simulink model "FOCandPMSM"  (R2022b)
settings: Solver=FixedStepAuto  StartTime=0.0  StopTime=inf  RelTol=1e-3  EnableMultiTasking=on
PreLoadFcn:
  | Ts = 1e-4;
  | Tcpu = 50e-6; %Controller sample time
  | 
  | % PMSM parameters
  | PM = 0.03; % Permanent magnet flux linkage
  | Ld = 2e-4;  % d-axis inductance
  | Lq = 2e-4;  % q-axis inductance
  | L0 = 2e-4;  % 0-axis inductance
  | Rs = 0.013; % Stator resistance
  | N = 6; % Number of pole pairs
  | J = 0.2; % Moment of inertia
  | 
  | % encoder parameters
  | numSlits = 2000; % number of slits
  | pulseSigOffset = 0; % index pulse signal offset
  | shaftInitPos = 0; % motor shaft initial position
  | 
  | % DAC parameters
  | gain = 0.1;
  | bias = 0;
  | 
  | % circuit parameters
  | Vdc = 48;
  | 
  | % real-time parameters
  | ts_FPGA_clk = 5e-9;
  | ts_FPGA_mdl = 1e-6;
  | 
  | % Real-time processor or embedded controller
  | RTorTTL = 1; % 1: Real-time processor,    0: embedded controller
  | 
  | % sample times
  | f_base = 200e6;
  | PWM_frequency = 20e3;
  | ts_FPGA_clk = 1/f_base;
  | ts_FPGA_mdl =1e-6;
  | 
  | PMSM_HIL_Param;
values from neighbouring files (symbols this model uses):
  inverter = mcb_updateInverterParameters(pmsm,inverter,target)    [embedded_sim_codegen_data.m]
  pmsm = mcb_SetPMSMMotorParameters('Teknic2310P')    [embedded_sim_codegen_data.m]
  PU_System = mcb_SetPUSystem(pmsm,inverter)    [embedded_sim_codegen_data.m]
  SpeedRef = 1    [PMSM_HIL_Param.m]
  T_cpu = T_pwm    (= 5e-05)    [embedded_sim_codegen_data.m]
  Tsw = 1/f_sw    [PMSM_HIL_Param.m]
undefined symbols (not defined in the file or in its folder): IO334
libraries: speedgoatlib_hdlCoder_IO3xx x28, mcbpositiondecoderlib x2, mcbhdlplantlib x1, slrtencoderlib x1, slrtresolverlib x1, mcbcontrolslib x1
settings Model: Creator=chrisz  LastModifiedBy=chrisz
settings SolverCC: ConcurrentTasks=on  PositivePriorityOrder=on
settings OptimizationCC: BlockReduction=off  ConditionallyExecuteInputs=off  OptimizeBlockIOStorage=off
settings DebuggingCC: AlgebraicLoopMsg=error  InheritedTsInSrcMsg=none  SingleTaskRateTransMsg=error  TasksWithSamePriorityMsg=none  ParameterOverflowMsg=none  ParameterUnderflowMsg=error  ParameterPrecisionLossMsg=none  InheritVATfromSVC=none  VariantConfigNotUsedByTopModel=none
settings HardwareCC: ProdBitPerLong=64  ProdLongLongMode=on  ProdHWDeviceType=Intel->x86-64 (Linux 64)  TargetBitPerPointer=64  TargetBitPerSizeT=64  TargetBitPerPtrDiffT=64  TargetLongLongMode=on  TargetIntDivRoundTo=Zero  TargetEndianess=LittleEndian  TargetWordSize=64  TargetHWDeviceType=Custom Processor->MATLAB Host Computer
settings ModelReferenceCC: EnableRefExpFcnMdlSchedulingChecks=on
settings RTWCC: Description=Simulink Real-Time  SystemTargetFile=slrealtime.tlc  TemplateMakefile=slrealtime_default_tmf  Toolchain=Simulink Real-Time Toolchain  BuildConfiguration=Faster Runs  CodeExecutionProfiling=on  TargetLang=C++

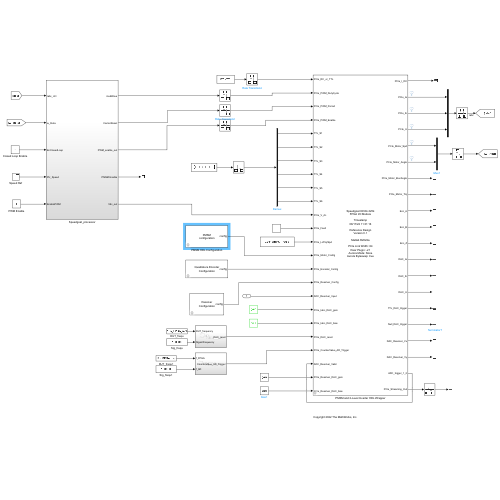
[thumbnail: Simulink's stored preview of the top-level diagram]
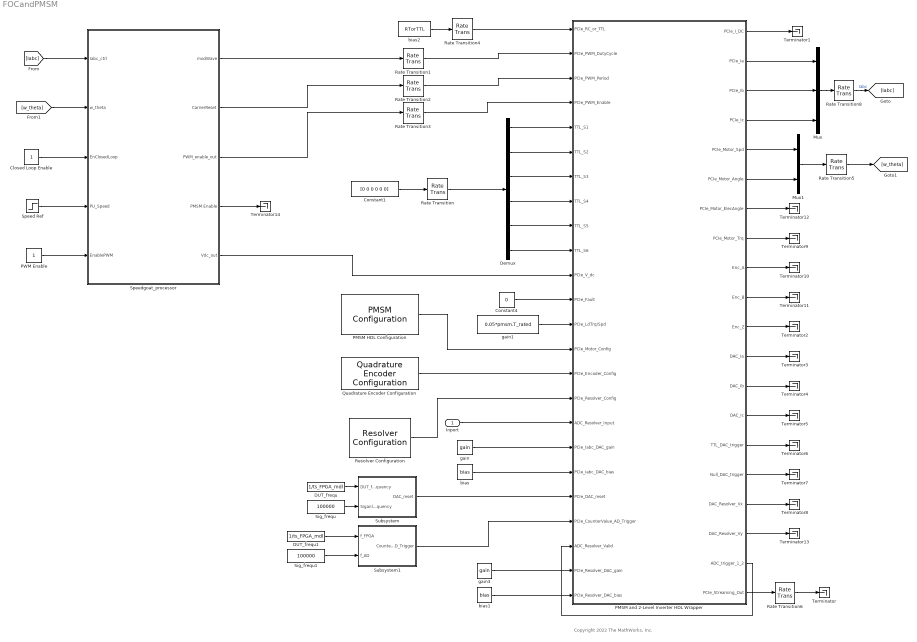
== system FOCandPMSM ==
  note: Copyright 2022 The MathWorks, Inc.
  Inport : Inport  OutDataTypeStr=int16
  Closed Loop Enable : Constant  OutDataTypeStr=Inherit: Inherit via back propagation  SampleTime=-1
  Constant1 : Constant  Value=[0 0 0 0 0 0]  OutDataTypeStr=boolean  SampleTime=-1
  Constant4 : Constant  Value=0  OutDataTypeStr=uint32  SampleTime=Tcpu
  DUT_frequ : Constant  Value=1/ts_FPGA_mdl  SampleTime=Tcpu
  DUT_frequ1 : Constant  Value=1/ts_FPGA_mdl  SampleTime=Tcpu
  Demux : Demux  Outputs=6
  Mux : Mux  Inputs=3
  Mux1 : Mux  Inputs=2
  PMSM HDL Configuration : mcbhdlplantlib/PMSM Configuration  portConfig=Torque  Trq_N_mode=0  Ts=Tcpu  Pp=pmsm.p  Rs=pmsm.Rs  Ld=pmsm.Ld  Lq=pmsm.Lq  lambda_pm=pmsm.FluxPM  J=pmsm.J  B=pmsm.B  f=0
      settings: LibrarySourceBlock=mcbhdllib/Electrical Systems/Motors/PMSM Configuration
  PMSM and 2-Level Inverter HDL Wrapper : Subsystem  mask(Speedgoat IO334-325k Interface Block){module_id=1, slot=-1, ts=-1, OutputRange=Auto (same as ADC), PullRPort0=pull-down, VioPort0=3.3V, PullRPort1=pull-down, VioPort1=3.3V, PullRPort2=pull-down, VioPort2=3.3V, PullRPort3=pull-down, VioPort3=3.3V, PullRPort4=pull-down, VioPort4=3.3V, PullRPort5=pull-down, VioPort5=3.3V, PullRPort6=pull-down, VioPort6=3.3V, FpgaFreq=200}
      mask prompts: module_id "FPGA Module Identifier:"; slot "PCI slot (-1: autosearch):"; ts "Sample time:"; OutputRange "DAC Voltage Range:"; PullRPort0 "pull resistor"; VioPort0 "I/O voltage"; PullRPort1 "pull resistor"; VioPort1 "I/O voltage"; PullRPort2 "pull resistor"; VioPort2 "I/O voltage"; PullRPort3 "pull resistor"; VioPort3 "I/O voltage"; PullRPort4 "pull resistor"; VioPort4 "I/O voltage"; PullRPort5 "pull resistor"; VioPort5 "I/O voltage"; PullRPort6 "pull resistor"; VioPort6 "I/O voltage"; FpgaFreq "FPGA Frequency [MHz]"
      mask help: Simulink Real-Time Interface Block for Speedgoat IO334-325k.
      mask init:
      | hdlslrt.backend.mfpgaparameters;
      mask Help: eval('speedgoatdoc_hdlc')
      mask TypeOptions OutputRange: IO334 DAC Setup/OutputRange
      mask TypeOptions PullRPort0: Port Settings -2x/PullRPort0
      mask Callback PullRPort0: sg_fpga_HDLCoder_io3xx_2x_m(2)
      mask TypeOptions VioPort0: Port Settings -2x/VioPort0
      mask Callback VioPort0: sg_fpga_HDLCoder_io3xx_2x_m(2)
      mask TypeOptions PullRPort1: Port Settings -2x/PullRPort1
      mask Callback PullRPort1: sg_fpga_HDLCoder_io3xx_2x_m(2)
      mask TypeOptions VioPort1: Port Settings -2x/VioPort1
      mask Callback VioPort1: sg_fpga_HDLCoder_io3xx_2x_m(2)
      mask TypeOptions PullRPort2: Port Settings -2x/PullRPort2
      mask Callback PullRPort2: sg_fpga_HDLCoder_io3xx_2x_m(2)
      mask TypeOptions VioPort2: Port Settings -2x/VioPort2
      mask Callback VioPort2: sg_fpga_HDLCoder_io3xx_2x_m(2)
      mask TypeOptions PullRPort3: Port Settings -2x/PullRPort3
      mask Callback PullRPort3: sg_fpga_HDLCoder_io3xx_2x_m(2)
      mask TypeOptions VioPort3: Port Settings -2x/VioPort3
      mask Callback VioPort3: sg_fpga_HDLCoder_io3xx_2x_m(2)
      mask TypeOptions PullRPort4: Port Settings -2x/PullRPort4
      mask Callback PullRPort4: sg_fpga_HDLCoder_io3xx_2x_m(2)
      mask TypeOptions VioPort4: Port Settings -2x/VioPort4
      mask Callback VioPort4: sg_fpga_HDLCoder_io3xx_2x_m(2)
      mask TypeOptions PullRPort5: Port Settings -2x/PullRPort5
      mask Callback PullRPort5: sg_fpga_HDLCoder_io3xx_2x_m(2)
      mask TypeOptions VioPort5: Port Settings -2x/VioPort5
      mask Callback VioPort5: sg_fpga_HDLCoder_io3xx_2x_m(2)
      mask TypeOptions PullRPort6: Port Settings -2x/PullRPort6
      mask Callback PullRPort6: sg_fpga_HDLCoder_io3xx_2x_m(2)
      mask TypeOptions VioPort6: Port Settings -2x/VioPort6
      mask Callback VioPort6: sg_fpga_HDLCoder_io3xx_2x_m(2)
      mask DialogControl AnalogOutput Prompt: Analog Output
      mask DialogControl IO33421 Prompt: IO334-21
      mask DialogControl port1 Prompt: Port 1
      mask DialogControl port2 Prompt: Port 2
      mask DialogControl port3 Prompt: Port 3
      mask DialogControl port4 Prompt: Port 4
      mask DialogControl port5 Prompt: Port 5
      mask DialogControl port6 Prompt: Port 6
      mask DialogControl port7 Prompt: Port 7
      mask Display:
      | SetupBlkPath = find_system(gcb, 'LookUnderMasks', 'all', 'FollowLinks', 'on', 'regexp', 'on', 'Name', 'IO3(\d|x){2}\s+Setup' );
      | SetupBlkPath = SetupBlkPath{1};
      | TS = get_param(SetupBlkPath,'timestamp_mcs');
      | disp(sprintf('Speedgoat IO334-325k\nFPGA I/O Module\n\nTimestamp\n%s\n\nReference Design\nVersion 0.1\n\nMatlab R2022a\n\nPCIe Link Width: X4\nRear Plugin: -21\nAurora Mode: None\nAurora Byteswap: true\n', TS))
  PWM Enable : Constant  OutDataTypeStr=Inherit: Inherit via back propagation  SampleTime=-1
  Quadrature Encoder Configuration : slrtencoderlib/Quadrature Encoder Configuration  NPulses=2000  zOffset=0  Ts=Tcpu
  Rate Transition{,1..6,8} (8 alike) : RateTransition  OutPortSampleTime=Tcpu
  Resolver Configuration : slrtresolverlib/Resolver Configuration  Ts=Tcpu  R=0.5  N=1  ADCrefV=5  ADCbits=16  totalADCCounts=65536
  Sig_frequ : Constant  Value=100000  VectorParams1D=off  SampleTime=Tcpu
  Sig_frequ1 : Constant  Value=100000  VectorParams1D=off  SampleTime=Tcpu
  Speed Ref : Step  Time=0.25  Before=1500/PU_System.N_base  After=SpeedRef  OutDataTypeStr=dataType  SampleTime=T_cpu
  Speedgoat_processor : Subsystem
  Subsystem : Subsystem
  Subsystem1 : Subsystem
  Terminator{,1..14} (15 alike) : Terminator
  bias : Constant  Value=bias  OutDataTypeStr=single  SampleTime=Tcpu
  bias1 : Constant  Value=bias  OutDataTypeStr=single  SampleTime=Tcpu
  bias2 : Constant  Value=RTorTTL  OutDataTypeStr=single  SampleTime=Tcpu
  gain : Constant  Value=gain  OutDataTypeStr=single  SampleTime=Tcpu
  gain1 : Constant  Value=0.05*pmsm.T_rated  OutDataTypeStr=single  SampleTime=Tcpu
  gain3 : Constant  Value=gain  OutDataTypeStr=single  SampleTime=Tcpu
  wires:
  bias1/1 -> PMSM and 2-Level Inverter HDL Wrapper/24(PCIe_Resolver_DAC_bias)
  gain3/1 -> PMSM and 2-Level Inverter HDL Wrapper/23(PCIe_Resolver_DAC_gain)
  Speedgoat_processor/1(modWave) -> Rate Transition1/1
  Rate Transition5/1 -> [w_theta]
  Mux1/1 -> Rate Transition5/1
  Rate Transition8/1 -> [Iabc]  "Iabc"
  Mux/1 -> Rate Transition8/1
  Rate Transition6/1 -> Terminator/1
  DUT_frequ1/1 -> Subsystem1/1(f_FPGA)
  Sig_frequ1/1 -> Subsystem1/2(f_AD)
  PMSM and 2-Level Inverter HDL Wrapper/19(ADC_trigger_1_2) -> PMSM and 2-Level Inverter HDL Wrapper/22(ADC_Resolver_Valid)
  Subsystem1/1(CounterValue_AD_Trigger) -> PMSM and 2-Level Inverter HDL Wrapper/21(PCIe_CounterValue_AD_Trigger)
  PMSM HDL Configuration/1 -> PMSM and 2-Level Inverter HDL Wrapper/14(PCIe_Motor_Config)
  Sig_frequ/1 -> Subsystem/2(SiganlFrequency)
  DUT_frequ/1 -> Subsystem/1(DUT_frequency)
  Constant1/1 -> Rate Transition/1
  Rate Transition/1 -> Demux/1
  bias2/1 -> Rate Transition4/1
  Speed Ref/1 -> Speedgoat_processor/4(PU_Speed)
  Closed Loop Enable/1 -> Speedgoat_processor/3(EnClosedLoop)
  PWM Enable/1 -> Speedgoat_processor/5(EnablePWM)
  [w_theta] -> Speedgoat_processor/2(w_theta)
  [Iabc] -> Speedgoat_processor/1(Iabc_ctrl)
  Speedgoat_processor/2(CarrierReset) -> Rate Transition2/1
  Speedgoat_processor/3(PWM_enable_out) -> Rate Transition3/1
  Speedgoat_processor/5(Vdc_out) -> PMSM and 2-Level Inverter HDL Wrapper/11(PCIe_V_dc)
  gain1/1 -> PMSM and 2-Level Inverter HDL Wrapper/13(PCIe_LdTrq/Spd)
  bias/1 -> PMSM and 2-Level Inverter HDL Wrapper/19(PCIe_Iabc_DAC_bias)
  Subsystem/1(DAC_reset) -> PMSM and 2-Level Inverter HDL Wrapper/20(PCIe_DAC_reset)
  Speedgoat_processor/4(PMSM Enable) -> Terminator14/1
  PMSM and 2-Level Inverter HDL Wrapper/20(PCIe_Streaming_Out) -> Rate Transition6/1
  PMSM and 2-Level Inverter HDL Wrapper/18(DAC_Resolver_Vy) -> Terminator13/1
  PMSM and 2-Level Inverter HDL Wrapper/17(DAC_Resolver_Vx) -> Terminator8/1
  PMSM and 2-Level Inverter HDL Wrapper/16(Null_DAC_trigger) -> Terminator7/1
  PMSM and 2-Level Inverter HDL Wrapper/15(TTL_DAC_trigger) -> Terminator6/1
  PMSM and 2-Level Inverter HDL Wrapper/14(DAC_Ic) -> Terminator5/1
  PMSM and 2-Level Inverter HDL Wrapper/1(PCIe_I_DC) -> Terminator1/1
  PMSM and 2-Level Inverter HDL Wrapper/2(PCIe_Ia) -> Mux/1
  PMSM and 2-Level Inverter HDL Wrapper/3(PCIe_Ib) -> Mux/2
  PMSM and 2-Level Inverter HDL Wrapper/4(PCIe_Ic) -> Mux/3
  PMSM and 2-Level Inverter HDL Wrapper/5(PCIe_Motor_Spd) -> Mux1/1
  PMSM and 2-Level Inverter HDL Wrapper/6(PCIe_Motor_Angle) -> Mux1/2
  PMSM and 2-Level Inverter HDL Wrapper/7(PCIe_Motor_ElecAngle) -> Terminator12/1
  PMSM and 2-Level Inverter HDL Wrapper/8(PCIe_Motor_Trq) -> Terminator9/1
  PMSM and 2-Level Inverter HDL Wrapper/9(Enc_A) -> Terminator10/1
  PMSM and 2-Level Inverter HDL Wrapper/10(Enc_B) -> Terminator11/1
  PMSM and 2-Level Inverter HDL Wrapper/11(Enc_Z) -> Terminator2/1
  PMSM and 2-Level Inverter HDL Wrapper/12(DAC_Ia) -> Terminator3/1
  PMSM and 2-Level Inverter HDL Wrapper/13(DAC_Ib) -> Terminator4/1
  Rate Transition4/1 -> PMSM and 2-Level Inverter HDL Wrapper/1(PCIe_RC_or_TTL)
  Rate Transition1/1 -> PMSM and 2-Level Inverter HDL Wrapper/2(PCIe_PWM_DutyCycle)
  Rate Transition2/1 -> PMSM and 2-Level Inverter HDL Wrapper/3(PCIe_PWM_Period)
  Rate Transition3/1 -> PMSM and 2-Level Inverter HDL Wrapper/4(PCIe_PWM_Enable)
  Demux/1 -> PMSM and 2-Level Inverter HDL Wrapper/5(TTL_S1)
  Demux/2 -> PMSM and 2-Level Inverter HDL Wrapper/6(TTL_S2)
  Demux/3 -> PMSM and 2-Level Inverter HDL Wrapper/7(TTL_S3)
  Demux/4 -> PMSM and 2-Level Inverter HDL Wrapper/8(TTL_S4)
  Demux/5 -> PMSM and 2-Level Inverter HDL Wrapper/9(TTL_S5)
  Demux/6 -> PMSM and 2-Level Inverter HDL Wrapper/10(TTL_S6)
  Constant4/1 -> PMSM and 2-Level Inverter HDL Wrapper/12(PCIe_Fault)
  Quadrature Encoder Configuration/1 -> PMSM and 2-Level Inverter HDL Wrapper/15(PCIe_Encoder_Config)
  Resolver Configuration/1 -> PMSM and 2-Level Inverter HDL Wrapper/16(PCIe_Resolver_Config)
  Inport/1 -> PMSM and 2-Level Inverter HDL Wrapper/17(ADC_Resolver_Input)
  gain/1 -> PMSM and 2-Level Inverter HDL Wrapper/18(PCIe_Iabc_DAC_gain)

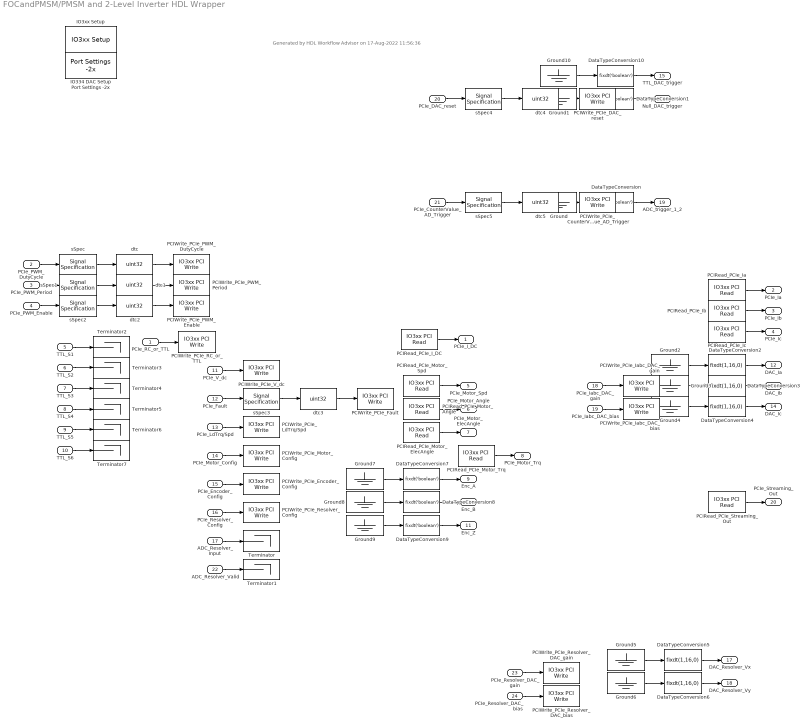
== system FOCandPMSM/PMSM and 2-Level Inverter HDL Wrapper ==
  note: Generated by HDL Workflow Advisor on 17-Aug-2022 11:56:36
  PCIe_RC_or_TTL : Inport
  PCIe_PWM_DutyCycle : Inport  Port=2
  PCIe_PWM_Period : Inport  Port=3
  PCIe_PWM_Enable : Inport  Port=4
  TTL_S1 : Inport  Port=5
  TTL_S2 : Inport  Port=6
  TTL_S3 : Inport  Port=7
  TTL_S4 : Inport  Port=8
  TTL_S5 : Inport  Port=9
  TTL_S6 : Inport  Port=10
  PCIe_V_dc : Inport  Port=11
  PCIe_Fault : Inport  Port=12
  PCIe_LdTrq/Spd : Inport  Port=13
  PCIe_Motor_Config : Inport  Port=14
  PCIe_Encoder_Config : Inport  Port=15
  PCIe_Resolver_Config : Inport  Port=16
  ADC_Resolver_Input : Inport  Port=17
  PCIe_Iabc_DAC_gain : Inport  Port=18
  PCIe_Iabc_DAC_bias : Inport  Port=19
  PCIe_DAC_reset : Inport  Port=20
  PCIe_CounterValue_AD_Trigger : Inport  Port=21  OutDataTypeStr=uint32
  ADC_Resolver_Valid : Inport  Port=22
  PCIe_Resolver_DAC_gain : Inport  Port=23
  PCIe_Resolver_DAC_bias : Inport  Port=24
  DataTypeConversion{,1,7..10} (6 alike) : DataTypeConversion  OutDataTypeStr=fixdt('boolean')  ConvertRealWorld=Stored Integer (SI)  SaturateOnIntegerOverflow=off  RndMeth=Floor
  DataTypeConversion{2..6} (5 alike) : DataTypeConversion  OutDataTypeStr=fixdt(1,16,0)  ConvertRealWorld=Stored Integer (SI)  SaturateOnIntegerOverflow=off  RndMeth=Floor
  Ground{,1..10} (11 alike) : Ground
  IO334 DAC Setup : speedgoatlib_hdlCoder_IO3xx/IO334 DAC Setup  module_id=module_id  OutputRange=Auto (same as ADC)
  IO3xx Setup : speedgoatlib_hdlCoder_IO3xx/IO3xx Setup  mdl_ss_name=slrt_pmsm_2level_inverterFrom22b/PMSM and 2-Level Inverter HDL Wrapper  board_type=IO334-325k  fpga_sync_mode=on  reset_mode=on  reset_mode_stop=off  device_id=1  module_id=module_id  pci_slot=slot  fpga_mat_file=hdl_prj\hdlsrc\slrt_pmsm_2level_inverterFrom22b\PMSMAnd2_LevelInverterHDLWrapper.mat  timestamp_mcs=08/17/22 11:31:16  timestamp=2208171019  tsreg=hex2dec('8')  bsf_file=PMSMAnd2_LevelInverterHDLWrapper.mcs  mcs=0
  PCIRead_PCIe_I_DC : speedgoatlib_hdlCoder_IO3xx/IO3xx PCI Read  device_id=1  module_id=module_id  board_type=IO334-325k  port_name=PCIe_I_DC  port_offset=hex2dec('184')  port_type=single  port_dim=1  strobe=0  sample_time=ts
  PCIRead_PCIe_Ia : speedgoatlib_hdlCoder_IO3xx/IO3xx PCI Read  device_id=1  module_id=module_id  board_type=IO334-325k  port_name=PCIe_Ia  port_offset=hex2dec('188')  port_type=single  port_dim=1  strobe=0  sample_time=ts
  PCIRead_PCIe_Ib : speedgoatlib_hdlCoder_IO3xx/IO3xx PCI Read  device_id=1  module_id=module_id  board_type=IO334-325k  port_name=PCIe_Ib  port_offset=hex2dec('18C')  port_type=single  port_dim=1  strobe=0  sample_time=ts
  PCIRead_PCIe_Ic : speedgoatlib_hdlCoder_IO3xx/IO3xx PCI Read  device_id=1  module_id=module_id  board_type=IO334-325k  port_name=PCIe_Ic  port_offset=hex2dec('1A4')  port_type=single  port_dim=1  strobe=0  sample_time=ts
  PCIRead_PCIe_Motor_Angle : speedgoatlib_hdlCoder_IO3xx/IO3xx PCI Read  device_id=1  module_id=module_id  board_type=IO334-325k  port_name=PCIe_Motor_Angle  port_offset=hex2dec('1AC')  port_type=single  port_dim=1  strobe=0  sample_time=ts
  PCIRead_PCIe_Motor_ElecAngle : speedgoatlib_hdlCoder_IO3xx/IO3xx PCI Read  device_id=1  module_id=module_id  board_type=IO334-325k  port_name=PCIe_Motor_ElecAngle  port_offset=hex2dec('1B0')  port_type=single  port_dim=1  strobe=0  sample_time=ts
  PCIRead_PCIe_Motor_Spd : speedgoatlib_hdlCoder_IO3xx/IO3xx PCI Read  device_id=1  module_id=module_id  board_type=IO334-325k  port_name=PCIe_Motor_Spd  port_offset=hex2dec('1A8')  port_type=single  port_dim=1  strobe=0  sample_time=ts
  PCIRead_PCIe_Motor_Trq : speedgoatlib_hdlCoder_IO3xx/IO3xx PCI Read  device_id=1  module_id=module_id  board_type=IO334-325k  port_name=PCIe_Motor_Trq  port_offset=hex2dec('124')  port_type=single  port_dim=1  strobe=0  sample_time=ts
  PCIRead_PCIe_Streaming_Out : speedgoatlib_hdlCoder_IO3xx/IO3xx PCI Read  device_id=1  module_id=module_id  board_type=IO334-325k  port_name=PCIe_Streaming_Out  port_offset=hex2dec('800')  port_type=single  port_dim=150  strobe=hex2dec('C00')  sample_time=ts
  PCIWrite_PCIe_CounterValue_AD_Trigger : speedgoatlib_hdlCoder_IO3xx/IO3xx PCI Write  device_id=1  module_id=module_id  board_type=IO334-325k  port_name=PCIe_CounterValue_AD_Trigger  port_offset=hex2dec('13C')  port_type=uint32  port_dim=1  strobe=0  sample_time=ts
  PCIWrite_PCIe_DAC_reset : speedgoatlib_hdlCoder_IO3xx/IO3xx PCI Write  device_id=1  module_id=module_id  board_type=IO334-325k  port_name=PCIe_DAC_reset  port_offset=hex2dec('138')  port_type=uint32  port_dim=1  strobe=0  sample_time=ts
  PCIWrite_PCIe_Encoder_Config : speedgoatlib_hdlCoder_IO3xx/IO3xx PCI Write  device_id=1  module_id=module_id  board_type=IO334-325k  port_name=PCIe_Encoder_Config  port_offset=hex2dec('190')  port_type=single  port_dim=3  strobe=hex2dec('1A0')  sample_time=ts
  PCIWrite_PCIe_Fault : speedgoatlib_hdlCoder_IO3xx/IO3xx PCI Write  device_id=1  module_id=module_id  board_type=IO334-325k  port_name=PCIe_Fault  port_offset=hex2dec('128')  port_type=uint32  port_dim=1  strobe=0  sample_time=ts
  PCIWrite_PCIe_Iabc_DAC_bias : speedgoatlib_hdlCoder_IO3xx/IO3xx PCI Write  device_id=1  module_id=module_id  board_type=IO334-325k  port_name=PCIe_Iabc_DAC_bias  port_offset=hex2dec('134')  port_type=single  port_dim=1  strobe=0  sample_time=ts
  PCIWrite_PCIe_Iabc_DAC_gain : speedgoatlib_hdlCoder_IO3xx/IO3xx PCI Write  device_id=1  module_id=module_id  board_type=IO334-325k  port_name=PCIe_Iabc_DAC_gain  port_offset=hex2dec('130')  port_type=single  port_dim=1  strobe=0  sample_time=ts
  PCIWrite_PCIe_LdTrq/Spd : speedgoatlib_hdlCoder_IO3xx/IO3xx PCI Write  device_id=1  module_id=module_id  board_type=IO334-325k  port_name=PCIe_LdTrq//Spd  port_offset=hex2dec('12C')  port_type=single  port_dim=1  strobe=0  sample_time=ts
  PCIWrite_PCIe_Motor_Config : speedgoatlib_hdlCoder_IO3xx/IO3xx PCI Write  device_id=1  module_id=module_id  board_type=IO334-325k  port_name=PCIe_Motor_Config  port_offset=hex2dec('140')  port_type=single  port_dim=9  strobe=hex2dec('180')  sample_time=ts
  PCIWrite_PCIe_PWM_DutyCycle : speedgoatlib_hdlCoder_IO3xx/IO3xx PCI Write  device_id=1  module_id=module_id  board_type=IO334-325k  port_name=PCIe_PWM_DutyCycle  port_offset=hex2dec('110')  port_type=uint32  port_dim=3  strobe=hex2dec('120')  sample_time=ts
  PCIWrite_PCIe_PWM_Enable : speedgoatlib_hdlCoder_IO3xx/IO3xx PCI Write  device_id=1  module_id=module_id  board_type=IO334-325k  port_name=PCIe_PWM_Enable  port_offset=hex2dec('108')  port_type=uint32  port_dim=1  strobe=0  sample_time=ts
  PCIWrite_PCIe_PWM_Period : speedgoatlib_hdlCoder_IO3xx/IO3xx PCI Write  device_id=1  module_id=module_id  board_type=IO334-325k  port_name=PCIe_PWM_Period  port_offset=hex2dec('104')  port_type=uint32  port_dim=1  strobe=0  sample_time=ts
  PCIWrite_PCIe_RC_or_TTL : speedgoatlib_hdlCoder_IO3xx/IO3xx PCI Write  device_id=1  module_id=module_id  board_type=IO334-325k  port_name=PCIe_RC_or_TTL  port_offset=hex2dec('100')  port_type=single  port_dim=1  strobe=0  sample_time=ts
  PCIWrite_PCIe_Resolver_Config : speedgoatlib_hdlCoder_IO3xx/IO3xx PCI Write  device_id=1  module_id=module_id  board_type=IO334-325k  port_name=PCIe_Resolver_Config  port_offset=hex2dec('1C0')  port_type=single  port_dim=6  strobe=hex2dec('1E0')  sample_time=ts
  PCIWrite_PCIe_Resolver_DAC_bias : speedgoatlib_hdlCoder_IO3xx/IO3xx PCI Write  device_id=1  module_id=module_id  board_type=IO334-325k  port_name=PCIe_Resolver_DAC_bias  port_offset=hex2dec('1B8')  port_type=single  port_dim=1  strobe=0  sample_time=ts
  PCIWrite_PCIe_Resolver_DAC_gain : speedgoatlib_hdlCoder_IO3xx/IO3xx PCI Write  device_id=1  module_id=module_id  board_type=IO334-325k  port_name=PCIe_Resolver_DAC_gain  port_offset=hex2dec('1B4')  port_type=single  port_dim=1  strobe=0  sample_time=ts
  PCIWrite_PCIe_V_dc : speedgoatlib_hdlCoder_IO3xx/IO3xx PCI Write  device_id=1  module_id=module_id  board_type=IO334-325k  port_name=PCIe_V_dc  port_offset=hex2dec('10C')  port_type=single  port_dim=1  strobe=0  sample_time=ts
  Port Settings -2x : speedgoatlib_hdlCoder_IO3xx/Port Settings -2x  module_id=module_id  rearIO=-21  PullRPort0=pull-down  VioPort0=3.3V  PullRPort1=pull-down  VioPort1=3.3V  PullRPort2=pull-down  VioPort2=3.3V  PullRPort3=pull-down  VioPort3=3.3V  PullRPort4=pull-down  VioPort4=3.3V  PullRPort5=pull-down  VioPort5=3.3V  PullRPort6=pull-down  VioPort6=3.3V
  Terminator{,1..7} (8 alike) : Terminator
  dtc{,1..5} (6 alike) : DataTypeConversion  OutDataTypeStr=uint32  ConvertRealWorld=Stored Integer (SI)  SaturateOnIntegerOverflow=off
  sSpec{,1,3,5} (4 alike) : SignalSpecification  OutDataTypeStr=fixdt(0,32,0)
  sSpec2 : SignalSpecification  OutDataTypeStr=fixdt('boolean')
  sSpec4 : SignalSpecification  OutDataTypeStr=fixdt(0,16,0)
  PCIe_I_DC : Outport
  PCIe_Ia : Outport  Port=2
  PCIe_Ib : Outport  Port=3
  PCIe_Ic : Outport  Port=4
  PCIe_Motor_Spd : Outport  Port=5
  PCIe_Motor_Angle : Outport  Port=6
  PCIe_Motor_ElecAngle : Outport  Port=7
  PCIe_Motor_Trq : Outport  Port=8
  Enc_A : Outport  Port=9
  Enc_B : Outport  Port=10
  Enc_Z : Outport  Port=11
  DAC_Ia : Outport  Port=12
  DAC_Ib : Outport  Port=13
  DAC_Ic : Outport  Port=14
  TTL_DAC_trigger : Outport  Port=15
  Null_DAC_trigger : Outport  Port=16
  DAC_Resolver_Vx : Outport  Port=17
  DAC_Resolver_Vy : Outport  Port=18
  ADC_trigger_1_2 : Outport  Port=19  OutDataTypeStr=boolean
  PCIe_Streaming_Out : Outport  Port=20
  wires:
  PCIe_RC_or_TTL/1 -> PCIWrite_PCIe_RC_or_TTL/1
  PCIe_PWM_DutyCycle/1 -> sSpec/1
  sSpec/1 -> dtc/1
  dtc/1 -> PCIWrite_PCIe_PWM_DutyCycle/1
  PCIe_PWM_Period/1 -> sSpec1/1
  sSpec1/1 -> dtc1/1
  dtc1/1 -> PCIWrite_PCIe_PWM_Period/1
  PCIe_PWM_Enable/1 -> sSpec2/1
  sSpec2/1 -> dtc2/1
  dtc2/1 -> PCIWrite_PCIe_PWM_Enable/1
  PCIe_V_dc/1 -> PCIWrite_PCIe_V_dc/1
  PCIe_Fault/1 -> sSpec3/1
  sSpec3/1 -> dtc3/1
  dtc3/1 -> PCIWrite_PCIe_Fault/1
  PCIe_LdTrq/Spd/1 -> PCIWrite_PCIe_LdTrq/Spd/1
  PCIe_Motor_Config/1 -> PCIWrite_PCIe_Motor_Config/1
  PCIe_Encoder_Config/1 -> PCIWrite_PCIe_Encoder_Config/1
  PCIe_Resolver_Config/1 -> PCIWrite_PCIe_Resolver_Config/1
  PCIe_Iabc_DAC_gain/1 -> PCIWrite_PCIe_Iabc_DAC_gain/1
  PCIe_Iabc_DAC_bias/1 -> PCIWrite_PCIe_Iabc_DAC_bias/1
  PCIe_DAC_reset/1 -> sSpec4/1
  sSpec4/1 -> dtc4/1
  dtc4/1 -> PCIWrite_PCIe_DAC_reset/1
  PCIe_CounterValue_AD_Trigger/1 -> sSpec5/1
  sSpec5/1 -> dtc5/1
  dtc5/1 -> PCIWrite_PCIe_CounterValue_AD_Trigger/1
  PCIe_Resolver_DAC_gain/1 -> PCIWrite_PCIe_Resolver_DAC_gain/1
  PCIe_Resolver_DAC_bias/1 -> PCIWrite_PCIe_Resolver_DAC_bias/1
  PCIRead_PCIe_I_DC/1 -> PCIe_I_DC/1
  PCIRead_PCIe_Ia/1 -> PCIe_Ia/1
  PCIRead_PCIe_Ib/1 -> PCIe_Ib/1
  PCIRead_PCIe_Ic/1 -> PCIe_Ic/1
  PCIRead_PCIe_Motor_Spd/1 -> PCIe_Motor_Spd/1
  PCIRead_PCIe_Motor_Angle/1 -> PCIe_Motor_Angle/1
  PCIRead_PCIe_Motor_ElecAngle/1 -> PCIe_Motor_ElecAngle/1
  PCIRead_PCIe_Motor_Trq/1 -> PCIe_Motor_Trq/1
  PCIRead_PCIe_Streaming_Out/1 -> PCIe_Streaming_Out/1
  ADC_Resolver_Input/1 -> Terminator/1
  ADC_Resolver_Valid/1 -> Terminator1/1
  DataTypeConversion/1 -> ADC_trigger_1_2/1
  Ground/1 -> DataTypeConversion/1
  DataTypeConversion1/1 -> Null_DAC_trigger/1
  Ground1/1 -> DataTypeConversion1/1
  DataTypeConversion2/1 -> DAC_Ia/1
  Ground2/1 -> DataTypeConversion2/1
  DataTypeConversion3/1 -> DAC_Ib/1
  Ground3/1 -> DataTypeConversion3/1
  DataTypeConversion4/1 -> DAC_Ic/1
  Ground4/1 -> DataTypeConversion4/1
  DataTypeConversion5/1 -> DAC_Resolver_Vx/1
  Ground5/1 -> DataTypeConversion5/1
  DataTypeConversion6/1 -> DAC_Resolver_Vy/1
  Ground6/1 -> DataTypeConversion6/1
  TTL_S1/1 -> Terminator2/1
  TTL_S2/1 -> Terminator3/1
  TTL_S3/1 -> Terminator4/1
  TTL_S4/1 -> Terminator5/1
  TTL_S5/1 -> Terminator6/1
  TTL_S6/1 -> Terminator7/1
  DataTypeConversion7/1 -> Enc_A/1
  Ground7/1 -> DataTypeConversion7/1
  DataTypeConversion8/1 -> Enc_B/1
  Ground8/1 -> DataTypeConversion8/1
  DataTypeConversion9/1 -> Enc_Z/1
  Ground9/1 -> DataTypeConversion9/1
  DataTypeConversion10/1 -> TTL_DAC_trigger/1
  Ground10/1 -> DataTypeConversion10/1

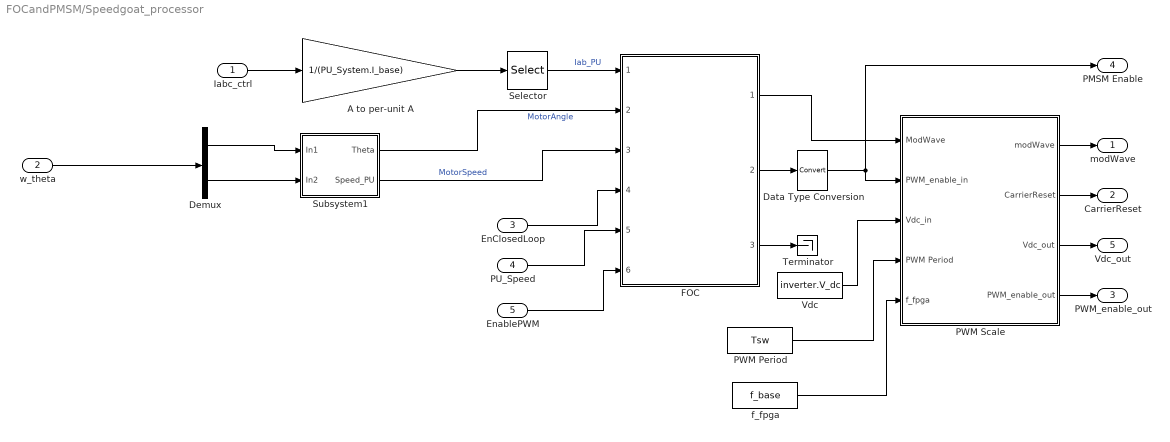
== system FOCandPMSM/Speedgoat_processor ==
  Iabc_ctrl : Inport
  w_theta : Inport  Port=2
  EnClosedLoop : Inport  Port=3
  PU_Speed : Inport  Port=4
  EnablePWM : Inport  Port=5
  A to per-unit A : Gain  Gain=1/(PU_System.I_base)
  Data Type Conversion : DataTypeConversion  SaturateOnIntegerOverflow=off  RndMeth=Floor
  Demux : Demux  Outputs=2
  FOC : Subsystem  ReferencedSubsystem=Field_Oriented_Control  AxisAlignment=D-axis
  PWM Period : Constant  Value=Tsw  SampleTime=-1
  PWM Scale : Subsystem
  Selector : Selector  InputPortWidth=3  IndexOptions=Index vector (dialog)  Indices=[1 2]  OutputSizes=1
  Subsystem1 : Subsystem
  Terminator : Terminator
  Vdc : Constant  Value=inverter.V_dc  OutDataTypeStr=single  SampleTime=T_cpu
  f_fpga : Constant  Value=f_base  SampleTime=-1
  modWave : Outport
  CarrierReset : Outport  Port=2
  PWM_enable_out : Outport  Port=3
  PMSM Enable : Outport  Port=4
  Vdc_out : Outport  Port=5
  wires:
  Data Type Conversion/1 -> PMSM Enable/1, PWM Scale/2(PWM_enable_in)
  f_fpga/1 -> PWM Scale/5(f_fpga)
  PWM Period/1 -> PWM Scale/4(PWM Period)
  Vdc/1 -> PWM Scale/3(Vdc_in)
  Subsystem1/1(Theta) -> FOC/2  "MotorAngle"
  FOC/3 -> Terminator/1
  FOC/2 -> Data Type Conversion/1
  Demux/2 -> Subsystem1/2(In2)
  Subsystem1/2(Speed_PU) -> FOC/3  "MotorSpeed"
  Iabc_ctrl/1 -> A to per-unit A/1
  Demux/1 -> Subsystem1/1(In1)
  A to per-unit A/1 -> Selector/1
  FOC/1 -> PWM Scale/1(ModWave)
  PWM Scale/3(Vdc_out) -> Vdc_out/1
  Selector/1 -> FOC/1  "Iab_PU"
  w_theta/1 -> Demux/1
  EnablePWM/1 -> FOC/6
  PU_Speed/1 -> FOC/5
  PWM Scale/2(CarrierReset) -> CarrierReset/1
  PWM Scale/4(PWM_enable_out) -> PWM_enable_out/1
  EnClosedLoop/1 -> FOC/4
  PWM Scale/1(modWave) -> modWave/1

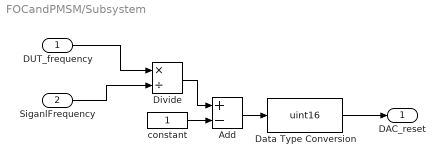
== system FOCandPMSM/Subsystem ==
  DUT_frequency : Inport
  SiganlFrequency : Inport  Port=2
  Add : Sum  Inputs=+-
  Data Type Conversion : DataTypeConversion  OutDataTypeStr=uint16  SaturateOnIntegerOverflow=off  RndMeth=Floor
  Divide : Product  Inputs=*/
  constant : Constant  VectorParams1D=off  SampleTime=-1
  DAC_reset : Outport
  wires:
  SiganlFrequency/1 -> Divide/2
  Add/1 -> Data Type Conversion/1
  Divide/1 -> Add/1
  Data Type Conversion/1 -> DAC_reset/1
  constant/1 -> Add/2
  DUT_frequency/1 -> Divide/1

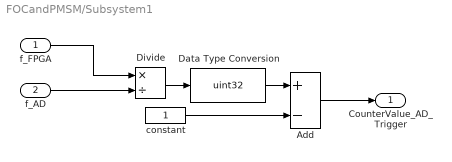
== system FOCandPMSM/Subsystem1 ==
  f_FPGA : Inport
  f_AD : Inport  Port=2
  Add : Sum  Inputs=+-  AccumDataTypeStr=uint32
  Data Type Conversion : DataTypeConversion  OutDataTypeStr=uint32  SaturateOnIntegerOverflow=off  RndMeth=Floor
  Divide : Product  Inputs=*/
  constant : Constant  VectorParams1D=off  OutDataTypeStr=uint32  SampleTime=-1
  CounterValue_AD_Trigger : Outport
  wires:
  Add/1 -> CounterValue_AD_Trigger/1
  constant/1 -> Add/2
  Data Type Conversion/1 -> Add/1
  Divide/1 -> Data Type Conversion/1
  f_FPGA/1 -> Divide/1
  f_AD/1 -> Divide/2

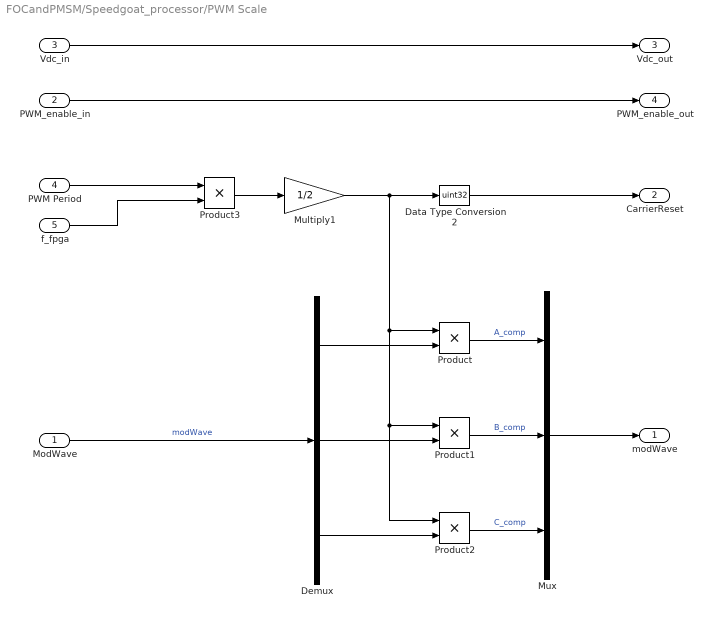
== system FOCandPMSM/Speedgoat_processor/PWM Scale ==
  ModWave : Inport
  PWM_enable_in : Inport  Port=2
  Vdc_in : Inport  Port=3
  PWM Period : Inport  Port=4
  f_fpga : Inport  Port=5
  Data Type Conversion2 : DataTypeConversion  OutDataTypeStr=uint32  SaturateOnIntegerOverflow=off  RndMeth=Floor
  Demux : Demux  Outputs=3
  Multiply1 : Gain  Gain=1/2
  Mux : Mux  Inputs=3
  Product : Product  OutDataTypeStr=uint32
  Product1 : Product  OutDataTypeStr=uint32
  Product2 : Product  OutDataTypeStr=uint32
  Product3 : Product
  modWave : Outport  VectorParamsAs1DForOutWhenUnconnected=off
  CarrierReset : Outport  Port=2  VectorParamsAs1DForOutWhenUnconnected=off
  Vdc_out : Outport  Port=3  VectorParamsAs1DForOutWhenUnconnected=off
  PWM_enable_out : Outport  Port=4  VectorParamsAs1DForOutWhenUnconnected=off
  wires:
  ModWave/1 -> Demux/1  "modWave"
  Multiply1/1 -> Product2/1, Product1/1, Product/1, Data Type Conversion2/1
  PWM Period/1 -> Product3/1
  Data Type Conversion2/1 -> CarrierReset/1
  Demux/1 -> Product/2
  Demux/2 -> Product1/2
  Demux/3 -> Product2/2
  f_fpga/1 -> Product3/2
  Product3/1 -> Multiply1/1
  Product1/1 -> Mux/2  "B_comp"
  Product/1 -> Mux/1  "A_comp"
  Product2/1 -> Mux/3  "C_comp"
  Vdc_in/1 -> Vdc_out/1
  PWM_enable_in/1 -> PWM_enable_out/1
  Mux/1 -> modWave/1

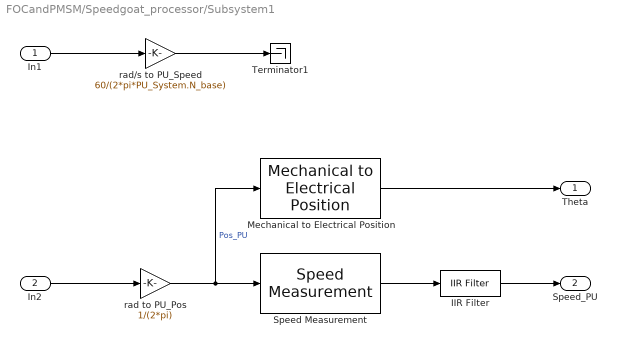
== system FOCandPMSM/Speedgoat_processor/Subsystem1 ==
  In1 : Inport
  In2 : Inport  Port=2
  IIR Filter : mcbcontrolslib/IIR Filter  VariantControl=Low Pass Filter  VariantSelect=Low-pass  Filter_constant=0.01  advancedSettings=off  Ts=50e-6  cutOff_freq=32.1525
  Mechanical to Electrical Position : mcbpositiondecoderlib/Mechanical to Electrical Position  NrPP=pmsm.p  selectedRange=Per unit  MechOfstInputType=Specify via dialog  mechOffsetIn=0  maxAngleIn=1  InputDataType=single  VariantSelect=floating-point
  Speed Measurement : mcbpositiondecoderlib/Speed Measurement  PositionUnit=Per unit  PositionScalingDatatype=uint32  SpeedCalculationMode=Time interval for speed calculation  SampleTimeAsync=T_cpu  MaximumApplicationSpeed=6000  SpeedResolution=5e-6  DelayLength=20  MaximumMeasurableSpeed=29999  MeasurableSpeedResolution=1.397e-05  SpeedUnit=Per unit based on dialog  PerUnitSpeed=PU_System.N_base  SpeedDataType=dataType
  Terminator1 : Terminator
  rad to PU_Pos : Gain  Gain=1/(2*pi)
  rad/s to PU_Speed : Gain  Gain=60/(2*pi*PU_System.N_base)
  Theta : Outport
  Speed_PU : Outport  Port=2
  wires:
  In1/1 -> rad/s to PU_Speed/1
  Speed Measurement/1 -> IIR Filter/1
  In2/1 -> rad to PU_Pos/1
  Mechanical to Electrical Position/1 -> Theta/1
  IIR Filter/1 -> Speed_PU/1
  rad to PU_Pos/1 -> Speed Measurement/1, Mechanical to Electrical Position/1  "Pos_PU"
  rad/s to PU_Speed/1 -> Terminator1/1
